simulink model "MotroCycleExperiment"  (R2023b)
settings: Solver=FixedStepAuto  StartTime=0.0  StopTime=inf  RelTol=1e-3  EnableMultiTasking=on
libraries: arduinomotorcarrierlib x4, simulink x1, eeGeneralControl x1, arduinosensorlib x1
settings Model: SimulationMode=external  ExtModeTrigDuration=2  Creator=bkhusain  LastModifiedBy=root
settings SolverCC: AlgebraicLoopSolver=TrustRegion
settings OptimizationCC: EnhancedBackFolding=on  PassReuseOutputArgsAs=Individual arguments  ZeroExternalMemoryAtStartup=off  ZeroInternalMemoryAtStartup=off  MaxStackSize=64  OptimizeBlockOrder=speed  DifferentSizesBufferReuse=on  OptimizationCustomize=off  EfficientTunableParamExpr=on
settings DebuggingCC: ParameterTunabilityLossMsg=error  UnconnectedInputMsg=warning  UnconnectedOutputMsg=warning  UnconnectedLineMsg=warning
settings HardwareCC: ProdBitPerPointer=32  ProdBitPerSizeT=32  ProdBitPerPtrDiffT=32  ProdLargestAtomicInteger=Long  ProdLargestAtomicFloat=Double  ProdWordSize=32  ProdHWDeviceType=ARM Compatible->ARM Cortex
settings ModelReferenceCC: EnableRefExpFcnMdlSchedulingChecks=on
settings SFSimCC: MATLABDynamicMemAlloc=off
settings RTWCC: Description=Embedded Coder  SystemTargetFile=ert.tlc  HardwareBoard=Arduino Nano 33 IoT  TemplateMakefile=ert_default_tmf  Toolchain=Arduino ARM  BuildConfiguration=Faster Runs
settings CodeAppCC: ForceParamTrailComments=on  IgnoreCustomStorageClasses=off  OperatorAnnotations=on  SimulinkDataObjDesc=on  SFDataObjDesc=on  InsertBlockDesc=on
settings ERTTargetCC: SupportContinuousTime=on  SupportVariableSizeSignals=on  ExtModeStaticAllocSize=8192

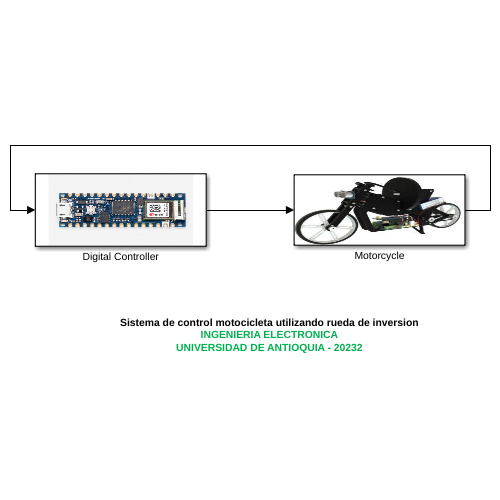
[thumbnail: Simulink's stored preview of the top-level diagram]
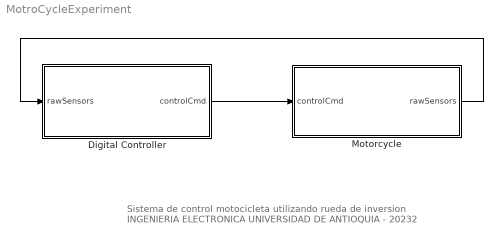
== system MotroCycleExperiment ==
  note: Sistema de control motocicleta utilizando rueda de inversion
      | INGENIERIA ELECTRONICA
      | UNIVERSIDAD DE ANTIOQUIA - 20232
  Digital Controller : Subsystem
      mask Display: image('arduinoNano.png'); % Use "Edit Image" on toolstrip to change.
  Motorcycle : Subsystem
      mask Display: image('motorcycle.jpg'); % Use "Edit Image" on toolstrip to change.
  wires:
  Digital Controller/1(controlCmd) -> Motorcycle/1(controlCmd)
  Motorcycle/1(rawSensors) -> Digital Controller/1(rawSensors)

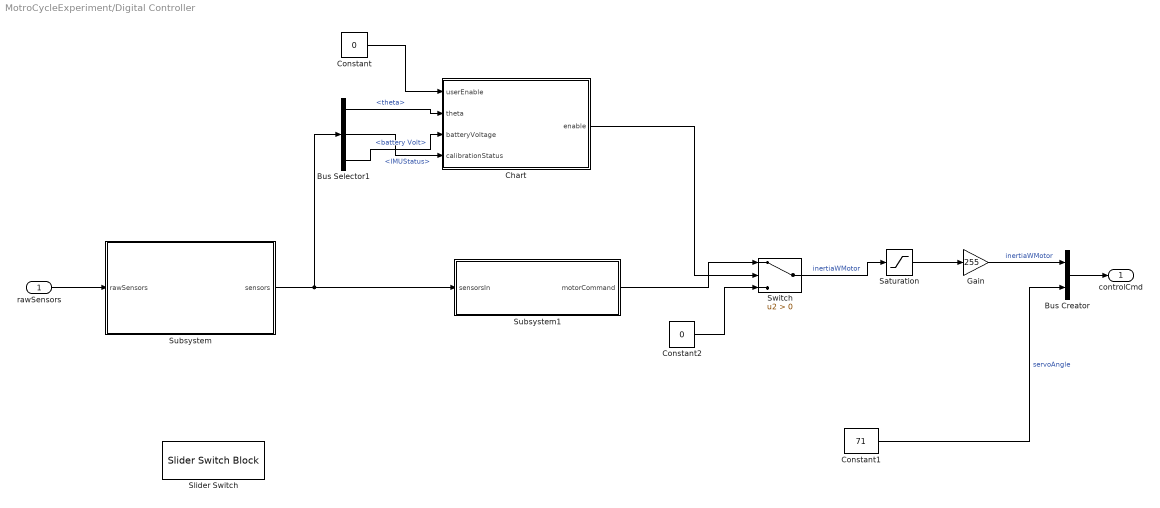
== system MotroCycleExperiment/Digital Controller ==
  rawSensors : Inport
  Bus Creator : BusCreator  Inputs=2
  Bus Selector1 : BusSelector  OutputSignals=theta,IMUStatus,battery Volt
  Chart : Stateflow chart  TreatAsAtomicUnit=on
  Constant : Constant  Value=0
  Constant1 : Constant  Value=71  SampleTime=0.01
  Constant2 : Constant  Value=0  SampleTime=0.01
  Gain : Gain  Gain=255
  Saturation : Saturate  UpperLimit=1  LowerLimit=-1
  Slider Switch : SliderSwitchBlock
      settings: Values={{'Off', 'On'}, [0 1]}
  Subsystem : Subsystem
  Subsystem1 : Subsystem
  Switch : Switch  Criteria=u2 > Threshold  SaturateOnIntegerOverflow=off  InputSameDT=off
  controlCmd : Outport
  wires:
  Bus Creator/1 -> controlCmd/1
  Switch/1 -> Saturation/1  "inertiaWMotor"
  rawSensors/1 -> Subsystem/1(rawSensors)
  Subsystem/1(sensors) -> Bus Selector1/1, Subsystem1/1(sensorsIn)
  Constant2/1 -> Switch/3
  Chart/1(enable) -> Switch/2
  Constant/1 -> Chart/1(userEnable)
  Bus Selector1/1 -> Chart/2(theta)  "<theta>"
  Bus Selector1/2 -> Chart/4(calibrationStatus)  "<IMUStatus>"
  Bus Selector1/3 -> Chart/3(batteryVoltage)  "<battery Volt>"
  Subsystem1/1(motorCommand) -> Switch/1
  Constant1/1 -> Bus Creator/2  "servoAngle"
  Saturation/1 -> Gain/1
  Gain/1 -> Bus Creator/1  "inertiaWMotor"

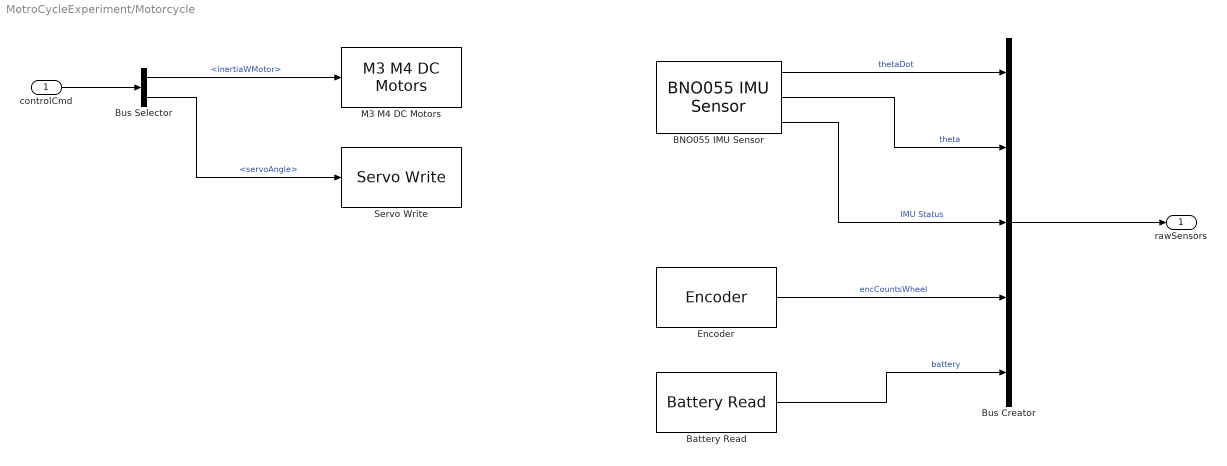
== system MotroCycleExperiment/Motorcycle ==
  controlCmd : Inport
  BNO055 IMU Sensor : arduinosensorlib/BNO055 IMU Sensor  SlaveAddress=0x28  OperationMode=Fusion  Accel=off  AngularRate=on  MagField=off  EulerAngles=on  Quat=off  LinearAccel=off  GravityVector=off  Status=on  Timestamp=off  AccelRange=4G  AccelBW=62.5 Hz  GyroRange=2000 dps  GyroBW=32 Hz  MagODR=10 Hz  spf=1  SampleTime=0.01  blockPlatform=ARDUINO  QueueSizeFactor=1
  Battery Read : arduinomotorcarrierlib/Battery Read  SlaveAddress=uint8( hex2dec( '66' ) )  blockPlatform=ARDUINO  SampleTime=0.01
  Bus Creator : BusCreator  Inputs=5
  Bus Selector : BusSelector  OutputSignals=inertiaWMotor,servoAngle
  Encoder : arduinomotorcarrierlib/Encoder  SlaveAddress=uint8( hex2dec( '66' ) )  blockPlatform=ARDUINO  Encoder=1  ShowSpeed=off  ResetOption=on  SampleTime=0.01
  M3 M4 DC Motors : arduinomotorcarrierlib/M3 M4 DC Motors  MotorNumber=M3  forwardPinNumber=3  reversePinNumber=2
  Servo Write : arduinomotorcarrierlib/Servo Write  SlaveAddress=uint8( hex2dec( '66' ) )  blockPlatform=ARDUINO  MotorNumber=3  MotorCarrierPWMFreq=100
  rawSensors : Outport
  wires:
  BNO055 IMU Sensor/1 -> Bus Creator/1  "thetaDot"
  BNO055 IMU Sensor/2 -> Bus Creator/2  "theta"
  BNO055 IMU Sensor/3 -> Bus Creator/3  "IMU Status"
  Encoder/1 -> Bus Creator/4  "encCountsWheel"
  Battery Read/1 -> Bus Creator/5  "battery"
  Bus Creator/1 -> rawSensors/1
  controlCmd/1 -> Bus Selector/1
  Bus Selector/2 -> Servo Write/1  "<servoAngle>"
  Bus Selector/1 -> M3 M4 DC Motors/1  "<inertiaWMotor>"

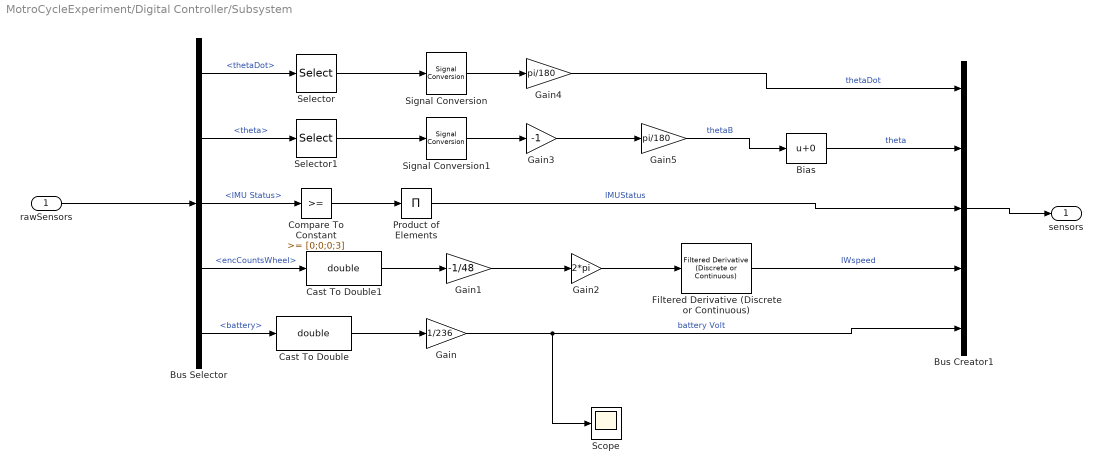
== system MotroCycleExperiment/Digital Controller/Subsystem ==
  rawSensors : Inport
  Bias : Bias  SaturateOnIntegerOverflow=off
  Bus Creator1 : BusCreator  Inputs=5
  Bus Selector : BusSelector  OutputSignals=thetaDot,theta,IMU Status,encCountsWheel,battery
  Cast To Double : DataTypeConversion  OutDataTypeStr=double  SaturateOnIntegerOverflow=off  RndMeth=Floor
  Cast To Double1 : DataTypeConversion  OutDataTypeStr=double  SaturateOnIntegerOverflow=off  RndMeth=Floor
  Compare To Constant : simulink/Logic and Bit Operations/Compare To Constant  relop=>=  const=[0;0;0;3]  OutDataTypeStr=boolean
  Filtered Derivative (Discrete or Continuous) : eeGeneralControl/Filtered Derivative (Discrete or Continuous)  K=1  T=0.1  B=inf  A=-inf  minRatio=10  init_option=Inherited from block input  x0=0  Ts=0.01
  Gain : Gain  Gain=1/236
  Gain1 : Gain  Gain=-1/48
  Gain2 : Gain  Gain=2*pi
  Gain3 : Gain  Gain=-1
  Gain4 : Gain  Gain=pi/180
  Gain5 : Gain  Gain=pi/180
  Product of Elements : Product  Inputs=*
  Scope : Scope
  Selector : Selector  InputPortWidth=3  IndexOptions=Index vector (dialog)  Indices=[2]  OutputSizes=1
  Selector1 : Selector  InputPortWidth=3  IndexOptions=Index vector (dialog)  Indices=[2]  OutputSizes=1
  Signal Conversion : SignalConversion  OverrideOpt=off
  Signal Conversion1 : SignalConversion  OverrideOpt=off
  sensors : Outport
  wires:
  Signal Conversion1/1 -> Gain3/1
  Product of Elements/1 -> Bus Creator1/3  "IMUStatus"
  Bus Selector/1 -> Selector/1  "<thetaDot>"
  Selector1/1 -> Signal Conversion1/1
  Gain1/1 -> Gain2/1
  Bus Selector/3 -> Compare To Constant/1  "<IMU Status>"
  Bus Creator1/1 -> sensors/1
  rawSensors/1 -> Bus Selector/1
  Cast To Double1/1 -> Gain1/1
  Selector/1 -> Signal Conversion/1
  Gain5/1 -> Bias/1  "thetaB"
  Filtered Derivative (Discrete or Continuous)/1 -> Bus Creator1/4  "IWspeed"
  Gain3/1 -> Gain5/1
  Bus Selector/2 -> Selector1/1  "<theta>"
  Bus Selector/4 -> Cast To Double1/1  "<encCountsWheel>"
  Cast To Double/1 -> Gain/1
  Bus Selector/5 -> Cast To Double/1  "<battery>"
  Gain/1 -> Scope/1, Bus Creator1/5  "battery Volt"
  Gain2/1 -> Filtered Derivative (Discrete or Continuous)/1
  Signal Conversion/1 -> Gain4/1
  Compare To Constant/1 -> Product of Elements/1
  Gain4/1 -> Bus Creator1/1  "thetaDot"
  Bias/1 -> Bus Creator1/2  "theta"

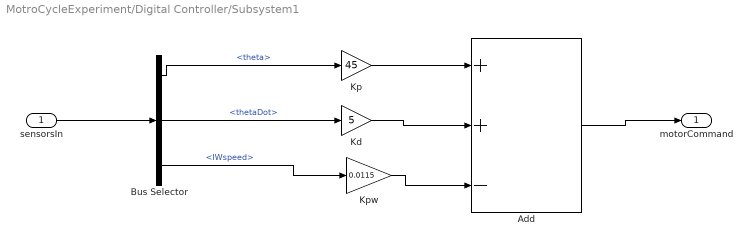
== system MotroCycleExperiment/Digital Controller/Subsystem1 ==
  sensorsIn : Inport
  Add : Sum  Inputs=++-
  Bus Selector : BusSelector  OutputSignals=theta,thetaDot,IWspeed
  Kd : Gain  Gain=5
  Kp : Gain  Gain=45
  Kpw : Gain  Gain=0.0115
  motorCommand : Outport
  wires:
  sensorsIn/1 -> Bus Selector/1
  Add/1 -> motorCommand/1
  Kpw/1 -> Add/3
  Kd/1 -> Add/2
  Kp/1 -> Add/1
  Bus Selector/1 -> Kp/1  "<theta>"
  Bus Selector/2 -> Kd/1  "<thetaDot>"
  Bus Selector/3 -> Kpw/1  "<IWspeed>"

== stateflow chart MotroCycleExperiment/Digital Controller/Chart ==
  state checkFallen [parallel]
    settings: executionOrder=1
    state Fallen
      entry: upright = false;
    state Standing
      entry: upright = true;
    (default) -> Fallen
    Fallen -> Standing : [abs(theta)<pi*12/180]
    Standing -> Fallen : [abs(theta) > pi*12/180]
  state checkIMUCalib [parallel]
    settings: executionOrder=2
    state imuNotCalibrated
      entry:
      IMUCalibrated = false;
    state imuCalibrated
      entry:
      IMUCalibrated = true;
    (default) -> imuNotCalibrated
    imuNotCalibrated -> imuCalibrated : [calibrationStatus == true]
  state checkBattery [parallel]
    settings: executionOrder=3
    state batteryNotCharged
      entry:
      batteryOK = false;
    state batteryCharged
      entry:
      batteryOK = true;
    (default) -> batteryNotCharged
    batteryNotCharged -> batteryCharged : [batteryVoltage > 3.2]
    batteryCharged -> batteryNotCharged : [batteryVoltage <= 3.2]
  state calculateEnable [parallel]
    settings: executionOrder=4
    state disableControl
      entry:
      enable = false
    state enableControl
      entry:
      enable = true
    (default) -> disableControl
    disableControl -> enableControl : [userEnable && batteryOK && IMUCalibrated && upright]
    enableControl -> disableControl : [not(userEnable) || not(batteryOK) || not(IMUCalibrated) || not(upright)]
  data: userEnable input; theta input; enable output; upright local; IMUCalibrated local; batteryOK local; batteryVoltage input; calibrationStatus input
